simulink model "Project-File"  (R2022b)
settings: Solver=VariableStepAuto  StartTime=0.0  StopTime=500  RelTol=1e-3
settings Model: Creator=shahm  LastModifiedBy=shahm

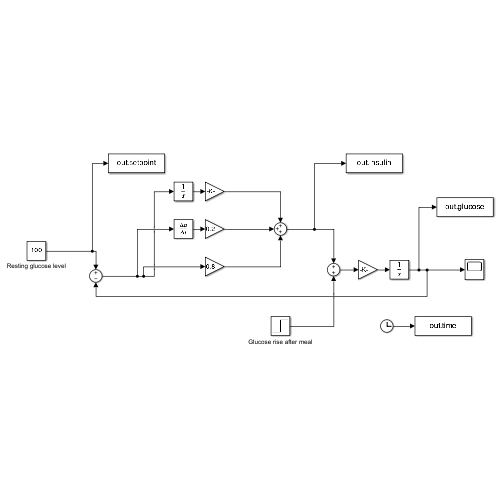
[thumbnail: Simulink's stored preview of the top-level diagram]
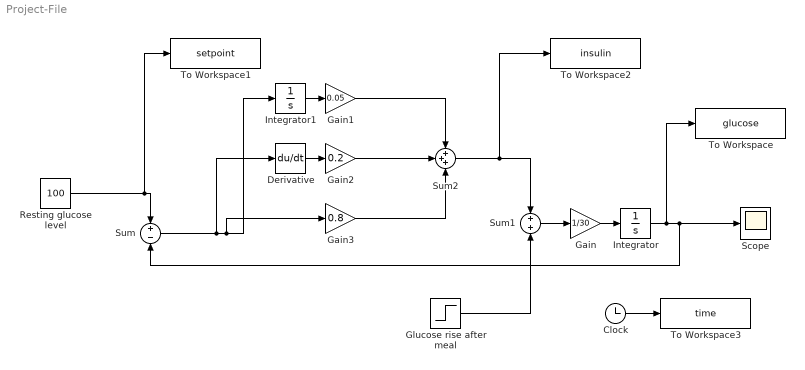
== system Project-File ==
  Clock : Clock
  Derivative : Derivative  CoefficientInTFapproximation=0.05
  Gain : Gain  Gain=1/30
  Gain1 : Gain  Gain=0.05
  Gain2 : Gain  Gain=0.2
  Gain3 : Gain  Gain=0.8
  Glucose rise after meal : Step  Time=20  After=100  SampleTime=0
  Integrator : Integrator  InitialCondition=100
  Integrator1 : Integrator
  Resting glucose level : Constant  Value=100
  Scope : Scope
  Sum : Sum  Inputs=+-
  Sum1 : Sum
  Sum2 : Sum  Inputs=+++
  To Workspace : ToWorkspace  VariableName=glucose  SampleTime=-1
  To Workspace1 : ToWorkspace  VariableName=setpoint  SampleTime=-1
  To Workspace2 : ToWorkspace  VariableName=insulin  SampleTime=-1
  To Workspace3 : ToWorkspace  VariableName=time  SampleTime=-1
  wires:
  Resting glucose level/1 -> To Workspace1/1, Sum/1
  Integrator/1 -> To Workspace/1, Scope/1, Sum/2
  Glucose rise after meal/1 -> Sum1/2
  Gain/1 -> Integrator/1
  Sum1/1 -> Gain/1
  Sum/1 -> Derivative/1, Gain3/1, Integrator1/1
  Integrator1/1 -> Gain1/1
  Gain1/1 -> Sum2/1
  Derivative/1 -> Gain2/1
  Gain2/1 -> Sum2/2
  Gain3/1 -> Sum2/3
  Sum2/1 -> To Workspace2/1, Sum1/1
  Clock/1 -> To Workspace3/1
